simulink library "windFrameToTangentialPlanePath_ul"  (R2018b)
settings: Solver=VariableStepAuto  StartTime=0.0  StopTime=10.0  RelTol=1e-3
values from neighbouring files (symbols this model uses):
  V = [-sin(phi1).*cos(lambda1), -sin(lambda1) ... (first row only)    [plotFigure8.m]
libraries: dspinverses x1
settings Model: Creator=James Reed  LastModifiedBy=James Reed

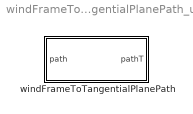
== system windFrameToTangentialPlanePath_ul ==
  windFrameToTangentialPlanePath : Subsystem

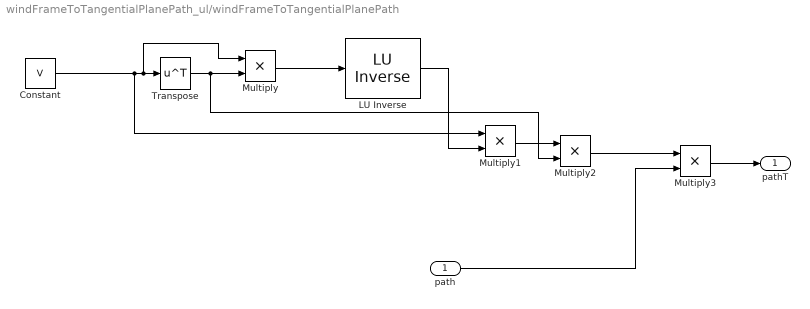
== system windFrameToTangentialPlanePath_ul/windFrameToTangentialPlanePath ==
  "path " : Inport
  " LU Inverse" : dspinverses/ LU Inverse
      settings: SourceProductName=DSP System Toolbox
  Constant : Constant  Value=V
  Multiply{,1..3} (4 alike) : Product
  Transpose : Math  Operator=transpose  SaturateOnIntegerOverflow=on
  pathT : Outport
  wires:
  Multiply/1 -> " LU Inverse"/1
  Transpose/1 -> Multiply2/2, Multiply/2
  "path "/1 -> Multiply3/2
  Multiply2/1 -> Multiply3/1
  Multiply1/1 -> Multiply2/1
  Constant/1 -> Multiply1/1, Multiply/1, Transpose/1
  Multiply3/1 -> pathT/1
  " LU Inverse"/1 -> Multiply1/2
